simulink model "s0415_R"  (Simulink 7.0)
settings: Solver=ode3  SolverMode=SingleTasking  StartTime=0.0  StopTime=900  FixedStep=1  MaxStep=1  RelTol=1e-3  AbsTol=1e-6
values from neighbouring files (symbols this model uses):
  Gsnen = Gs.den{1}    [m0404Bsp.m]
  Gszae = Gs.num{1}    [m0404Bsp.m]
  Kpr = 10    [m0108d.m]    (also in m0109b.m = 1; m0113c.m; m0404Bsp.m = 3)
  wdach_ = wdach    (= 1)    [m0404Bsp.m]
  zdach_ = zdach    (= 1)    [m0404Bsp.m]
undefined symbols (not defined in the file or in its folder): TB, Tn, ymax, ymin
settings Model: Creator=froriep  LastModifiedBy=froriep
settings DataIOCC: LimitDataPoints=off  SaveOutput=off  SaveTime=off
settings OptimizationCC: BooleanDataType=off
settings DebuggingCC: SaveWithParameterizedLinksMsg=none  SignalResolutionControl=TryResolveAllWithWarning  SolverPrmCheckMsg=none  MultiTaskDSMMsg=warning  MultiTaskCondExecSysMsg=none  StrictBusMsg=None
settings HardwareCC: TargetUnknown=on
settings RTWCC: IncludeERTFirstTime=on

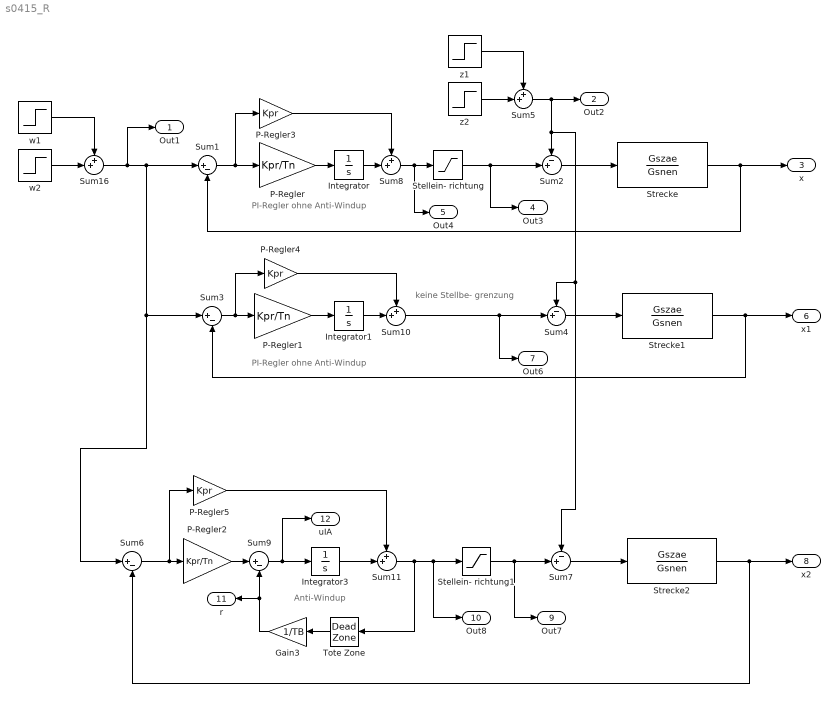
== system s0415_R ==
  note: PI-Regler
      | ohne Anti-Windup
  note: Anti-Windup
  note: PI-Regler
      | ohne Anti-Windup
  note: keine
      | Stellbe-
      | grenzung
  Gain3 : Gain  Orientation=left  Gain=1/TB  ParameterDataType=sfix(16)  ParameterScaling=2^0  OutDataType=sfix(16)  OutScaling=2^0
  Integrator : Integrator
  Integrator1 : Integrator
  Integrator3 : Integrator
  P-Regler : Gain  Gain=Kpr/Tn  ParameterDataType=sfix(16)  ParameterScaling=2^0  OutDataType=sfix(16)  OutScaling=2^0
  P-Regler1 : Gain  Gain=Kpr/Tn  ParameterDataType=sfix(16)  ParameterScaling=2^0  OutDataType=sfix(16)  OutScaling=2^0
  P-Regler2 : Gain  Gain=Kpr/Tn  ParameterDataType=sfix(16)  ParameterScaling=2^0  OutDataType=sfix(16)  OutScaling=2^0
  P-Regler3 : Gain  Gain=Kpr  ParameterDataType=sfix(16)  ParameterScaling=2^0  OutDataType=sfix(16)  OutScaling=2^0
  P-Regler4 : Gain  Gain=Kpr  ParameterDataType=sfix(16)  ParameterScaling=2^0  OutDataType=sfix(16)  OutScaling=2^0
  P-Regler5 : Gain  Gain=Kpr  ParameterDataType=sfix(16)  ParameterScaling=2^0  OutDataType=sfix(16)  OutScaling=2^0
  Stellein- richtung : Saturate  UpperLimit=ymax  LowerLimit=ymin  OutDataType=sfix(16)  OutScaling=2^0
  Stellein- richtung1 : Saturate  UpperLimit=ymax  LowerLimit=ymin  OutDataType=sfix(16)  OutScaling=2^0
  Strecke : TransferFcn  Numerator=Gszae  Denominator=Gsnen
  Strecke1 : TransferFcn  Numerator=Gszae  Denominator=Gsnen
  Strecke2 : TransferFcn  Numerator=Gszae  Denominator=Gsnen
  Sum1 : Sum  Inputs=|+-  SaturateOnIntegerOverflow=on  InputSameDT=on
  Sum10 : Sum  Inputs=++|  SaturateOnIntegerOverflow=on  InputSameDT=on
  Sum11 : Sum  Inputs=++|  SaturateOnIntegerOverflow=on  InputSameDT=on
  Sum16 : Sum  Inputs=++|  OutDataType=sfix(16)  OutScaling=2^0
  Sum2 : Sum  Inputs=-+|  SaturateOnIntegerOverflow=on  InputSameDT=on
  Sum3 : Sum  Inputs=|+-  SaturateOnIntegerOverflow=on  InputSameDT=on
  Sum4 : Sum  Inputs=-+|  SaturateOnIntegerOverflow=on  InputSameDT=on
  Sum5 : Sum  Inputs=++|  OutDataType=sfix(16)  OutScaling=2^0
  Sum6 : Sum  Inputs=|+-  SaturateOnIntegerOverflow=on  InputSameDT=on
  Sum7 : Sum  Inputs=-+|  SaturateOnIntegerOverflow=on  InputSameDT=on
  Sum8 : Sum  Inputs=++|  SaturateOnIntegerOverflow=on  InputSameDT=on
  Sum9 : Sum  Inputs=|+-  OutDataType=sfix(16)  OutScaling=2^0  SaturateOnIntegerOverflow=on  InputSameDT=on
  Tote Zone : DeadZone  Orientation=left  LowerValue=ymin  UpperValue=ymax  SaturateOnIntegerOverflow=on
  w1 : Step  After=wdach_  SampleTime=0
  w2 : Step  Time=11  After=-wdach_  SampleTime=0
  z1 : Step  After=zdach_  SampleTime=0
  z2 : Step  Time=11  After=-zdach_  SampleTime=0
  Out1 : Outport  OutDataType=sfix(16)  OutScaling=2^0
  Out2 : Outport  Port=2  OutDataType=sfix(16)  OutScaling=2^0
  x : Outport  Port=3  OutDataType=sfix(16)  OutScaling=2^0
  Out3 : Outport  Port=4  OutDataType=sfix(16)  OutScaling=2^0
  Out4 : Outport  Port=5  OutDataType=sfix(16)  OutScaling=2^0
  x1 : Outport  Port=6  OutDataType=sfix(16)  OutScaling=2^0
  Out6 : Outport  Port=7  OutDataType=sfix(16)  OutScaling=2^0
  x2 : Outport  Port=8  OutDataType=sfix(16)  OutScaling=2^0
  Out7 : Outport  Port=9  OutDataType=sfix(16)  OutScaling=2^0
  Out8 : Outport  Port=10  OutDataType=sfix(16)  OutScaling=2^0
  r : Outport  Orientation=left  Port=11  OutDataType=sfix(16)  OutScaling=2^0
  uIA : Outport  Port=12  OutDataType=sfix(16)  OutScaling=2^0
  wires:
  Sum5/1 -> Out2/1, Sum2/1, Sum4/1, Sum7/1
  Sum1/1 -> P-Regler/1, P-Regler3/1
  Strecke/1 -> Sum1/2, x/1
  Sum2/1 -> Strecke/1
  P-Regler/1 -> Integrator/1
  Stellein- richtung/1 -> Sum2/2, Out3/1
  Sum16/1 -> Out1/1, Sum1/1, Sum3/1, Sum6/1
  w2/1 -> Sum16/2
  w1/1 -> Sum16/1
  Sum3/1 -> P-Regler4/1, P-Regler1/1
  Strecke1/1 -> x1/1, Sum3/2
  Sum4/1 -> Strecke1/1
  P-Regler1/1 -> Integrator1/1
  z2/1 -> Sum5/2
  z1/1 -> Sum5/1
  Sum6/1 -> P-Regler5/1, P-Regler2/1
  Strecke2/1 -> x2/1, Sum6/2
  Sum7/1 -> Strecke2/1
  Stellein- richtung1/1 -> Out7/1, Sum7/2
  Sum9/1 -> uIA/1, Integrator3/1
  Tote Zone/1 -> Gain3/1
  Gain3/1 -> r/1, Sum9/2
  P-Regler3/1 -> Sum8/1
  Integrator/1 -> Sum8/2
  Sum8/1 -> Stellein- richtung/1, Out4/1
  Integrator1/1 -> Sum10/2
  Sum10/1 -> Sum4/2, Out6/1
  P-Regler4/1 -> Sum10/1
  Integrator3/1 -> Sum11/2
  P-Regler5/1 -> Sum11/1
  Sum11/1 -> Tote Zone/1, Stellein- richtung1/1, Out8/1
  P-Regler2/1 -> Sum9/1
